simulink model "zad1"  (Simulink 3.00)
settings: Solver=ode45  StartTime=0.0  StopTime=10.0  RelTol=1e-3
settings Model: LastModifiedBy=Administrator

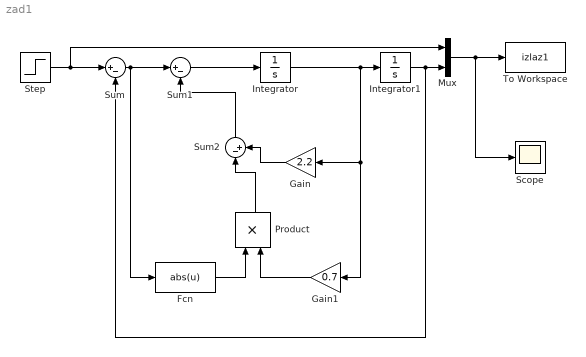
== system zad1 ==
  Fcn : Fcn  Expr=abs(u)
  Gain : Gain  Orientation=left  Gain=2.2  SaturateOnIntegerOverflow=on
  Gain1 : Gain  Orientation=left  Gain=0.7  SaturateOnIntegerOverflow=on
  Integrator : Integrator  ExternalReset=none  InitialConditionSource=internal  InitialCondition=0  LimitOutput=off  UpperSaturationLimit=inf  LowerSaturationLimit=-inf  ShowSaturationPort=off  ShowStatePort=off  AbsoluteTolerance=auto
  Integrator1 : Integrator  ExternalReset=none  InitialConditionSource=internal  InitialCondition=0  LimitOutput=off  UpperSaturationLimit=inf  LowerSaturationLimit=-inf  ShowSaturationPort=off  ShowStatePort=off  AbsoluteTolerance=auto
  Mux : Mux  Inputs=2
  Product : Product  Orientation=up  Inputs=2  SaturateOnIntegerOverflow=on
  Scope : Scope
      settings: TimeRange=auto  YMin=-5  YMax=5  SaveToWorkspace=off  SaveName=ScopeData
  Step : Step  Time=1  Before=0  After=3  SampleTime=0
  Sum : Sum  Inputs=|+-  SaturateOnIntegerOverflow=on
  Sum1 : Sum  Inputs=|+-  SaturateOnIntegerOverflow=on
  Sum2 : Sum  Orientation=up  Inputs=|-+  SaturateOnIntegerOverflow=on
  To Workspace : ToWorkspace  VariableName=izlaz1  SampleTime=-1  SaveFormat=Matrix
  wires:
  Sum1/1 -> Integrator/1
  Step/1 -> Sum/1, Mux/1
  Fcn/1 -> Product/1
  Gain1/1 -> Product/2
  Sum2/1 -> Sum1/2
  Gain/1 -> Sum2/2
  Product/1 -> Sum2/1
  Integrator/1 -> Integrator1/1, Gain1/1, Gain/1
  Sum/1 -> Sum1/1, Fcn/1
  Integrator1/1 -> Mux/2, Sum/2
  Mux/1 -> To Workspace/1, Scope/1
